simulink model "MIL4L3_SW6_V1_20220211"  (R2018b)
settings: Solver=FixedStepAuto  StartTime=0.0  StopTime=inf  FixedStep=0.001  RelTol=1e-3
PreLoadFcn:
  | A0_MILtest;
undefined symbols (not defined in the file or in its folder): Clb_ICADirect_LaneDisp_StateFive, Clb_ICADirect_LaneDisp_StateFour, Clb_ICADirect_LaneDisp_StateOne, Clb_ICADirect_LaneDisp_StateThree, Clb_ICADirect_LaneDisp_StateTwo, Clb_ICADirect_LaneDisp_StateZero, Clb_ICADirect_LaneDispSW, Clb_ICADirect_TrnLghtsCom_Switch, Clb_ICADirect_TrnLghtsCom_Value, Clb_ICADirect_TrnLghtsCrtl_Inhb, IMAP_Clb_ACU_Driver_Belt, IMAP_Clb_ACU_Driver_Belt_Over, IMAP_Clb_ACU_Passenger_Belt, IMAP_Clb_ACU_Passenger_Belt_Over, IMAP_Clb_ACU_RearLeft_Belt, IMAP_Clb_ACU_RearLeft_Belt_Over, IMAP_Clb_ACU_RearMiddle_Belt, IMAP_Clb_ACU_RearMiddle_Belt_Over, IMAP_Clb_ACU_RearRight_Belt, IMAP_Clb_ACU_RearRight_Belt_Over, IMAP_Clb_AEB_Switch, IMAP_Clb_AEB_Switch_Over, IMAP_Clb_ALC_TLC_Mode, IMAP_Clb_ALC_TLC_Mode_Over, IMAP_Clb_BCM_Battery_Voltage, IMAP_Clb_BCM_Battery_Voltage_Over, IMAP_Clb_BCM_BrakeLamp_State, IMAP_Clb_BCM_BrakeLamp_State_Over, IMAP_Clb_BCM_CHMSL_Status, IMAP_Clb_BCM_CHMSL_Status_Over, IMAP_Clb_BCM_Door_Lock_State, IMAP_Clb_BCM_Door_Lock_State_Over, IMAP_Clb_BCM_FrontWiper_State, IMAP_Clb_BCM_FrontWiper_State_Over, IMAP_Clb_BCM_FrontWiper_Switch, IMAP_Clb_BCM_FrontWiper_Switch_Over, IMAP_Clb_BCM_HazardLamp, IMAP_Clb_BCM_HazardLamp_Over, IMAP_Clb_BCM_HazardLamp_Switch, IMAP_Clb_BCM_HazardLamp_Switch_Over, IMAP_Clb_BCM_HighBeam_State, IMAP_Clb_BCM_HighBeam_State_Over, IMAP_Clb_BCM_Ignition_State, IMAP_Clb_BCM_Ignition_State_Over, IMAP_Clb_BCM_IHBC_Enabled, IMAP_Clb_BCM_IHBC_Enabled_Over, IMAP_Clb_BCM_Left_Light, IMAP_Clb_BCM_Left_Light_Over, IMAP_Clb_BCM_LeftTurn_Switch, IMAP_Clb_BCM_LeftTurn_Switch_Over, IMAP_Clb_BCM_LF_Door_State, IMAP_Clb_BCM_LF_Door_State_Over, IMAP_Clb_BCM_LowBeam_State, IMAP_Clb_BCM_LowBeam_State_Over, IMAP_Clb_BCM_LR_Door_State, IMAP_Clb_BCM_LR_Door_State_Over, IMAP_Clb_BCM_RF_Door_State, IMAP_Clb_BCM_RF_Door_State_Over, IMAP_Clb_BCM_Right_Light, IMAP_Clb_BCM_Right_Light_Over ... (+547)
libraries: CarMaker4SL x2153, simulink x292, dspstat3 x3, canmsglib x2, simulink_extras x1
(part 45 of 52)

== system MIL4L3_SW6_V1_20220211/CarMaker/VehicleControl/Function/LKA/LKAS1/LL/LLOn/LL State Determination (LLStateDet)/LL State Machine Conditions (LLSMCon)/Enable Condition (EnaC)/Vehicle State Condition (VehStateC) ==
  VehStateC_stDACMode : Inport
  VehStateC_bsInInfoSyn : Inport  Port=2
  VehStateC_bsLLClb : Inport  Port=3
  Bus Selector : BusSelector  OutputSignals=bsVehMovInfo.ESC_VehSpd,bsBCMInfo,bsPTState
  Bus Selector1 : BusSelector  OutputSignals=bsLLSMConClb.EnaCClb.LL_MAX_LDWS_SPEED_ENABLE,bsLLSMConClb.EnaCClb.LL_MAX_LKAS_SPEED_ENABLE,bsLLSMConClb.EnaCClb.LL_MIN_LKAS_SPEED_ENABLE
  Emergency Light Enable Condition (EmgcyLghtEC) : Subsystem  Description=|
      | Block Name: Emergency Light Enable Condition
      | Ab.: EmgcyLghtEC
      | No.: 1.1.1.2.1.3
      | Rev: 0.0.1
      | Update Date: 19-3-26
  Gear Enable Condition (GearEC) : Subsystem  Description=|
      | Block Name: Gear Enable Condition
      | Ab.: GearEC
      | No.: 1.1.1.2.1.4
      | Rev: 0.0.1
      | Update Date: 19-3-26
  Vehicle Speed Enable Condition (VehSpdEC) : Subsystem  Description=|
      | Block Name: Vehicle Speed Enable Condition
      | Ab.: VehSpdEC
      | No.: 1.1.1.2.1.1
      | Rev: 0.0.1
      | Update Date: 19-3-26
  Vehicle State Condition Synthesis (VehStateCSyn) : Subsystem  Description=|
      | Block Name: Vehicle State Condition Synthesis
      | Ab.: VehStateCSyn
      | No.: 1.1.1.2.1.5
      | Rev: 0.0.1
      | Update Date: 19-3-26
  VehStateC_stVehStateCSyn : Outport
  wires:
  Vehicle Speed Enable Condition (VehSpdEC)/1(VehSpdEC_stVehSpdECFlg) -> Vehicle State Condition Synthesis (VehStateCSyn)/1(VehStateCSyn_stVehSpdECFlg)  "VEHSTATE_VEHSPEED"
  VehStateC_bsInInfoSyn/1 -> Bus Selector/1
  Gear Enable Condition (GearEC)/1(GearEC_stGearECFlg) -> Vehicle State Condition Synthesis (VehStateCSyn)/3(VehStateCSyn_stGearECFlg)  "VEHSTATE_GEAR"
  Vehicle State Condition Synthesis (VehStateCSyn)/1(VehStateCSyn_stVehStateCSyn) -> VehStateC_stVehStateCSyn/1  "VEHSTATE"
  Bus Selector/1 -> Vehicle Speed Enable Condition (VehSpdEC)/2(VehSpdEC_vVehSpd)  "<ESC_VehSpd>"
  Bus Selector1/1 -> Vehicle Speed Enable Condition (VehSpdEC)/3(VehSpdEC_vLDWVehSpdMax_C)  "<LL_MAX_LDWS_SPEED_ENABLE>"
  Bus Selector1/3 -> Vehicle Speed Enable Condition (VehSpdEC)/5(VehSpdEC_vVehSpdMin_C)  "<LL_MIN_LKAS_SPEED_ENABLE>"
  Bus Selector1/2 -> Vehicle Speed Enable Condition (VehSpdEC)/4(VehSpdEC_vLKAVehSpdMax_C)  "<LL_MAX_LKAS_SPEED_ENABLE>"
  VehStateC_bsLLClb/1 -> Bus Selector1/1
  VehStateC_stDACMode/1 -> Vehicle Speed Enable Condition (VehSpdEC)/1(VehSpdEC_stDACMode)
  Bus Selector/3 -> Gear Enable Condition (GearEC)/1(GearEC_bsTCUState)  "<bsPTState>"
  Bus Selector/2 -> Emergency Light Enable Condition (EmgcyLghtEC)/1(EmgcyLghtEC_bsStLampState)  "<bsBCMInfo>"
  Emergency Light Enable Condition (EmgcyLghtEC)/1(EmgcyLghtEC_stEmgcyLghtECFlg) -> Vehicle State Condition Synthesis (VehStateCSyn)/2(VehStateCSyn_stEmgcyLghtECFlg)  "VEHSTATE_LIGHT"

== system MIL4L3_SW6_V1_20220211/CarMaker/VehicleControl/Function/LKA/LKAS1/LL/LLOn/LL State Determination (LLStateDet)/LL State Machine Conditions (LLSMCon)/Fault Condition (FaultC)/Count_5s1 ==
  SampleTime : Inport
  Enable : EnablePort  StatesWhenEnabling=reset
  Add : Sum
  Constant1 : Constant  Value=5  OutDataTypeStr=uint16
  Memory : Memory  InheritSampleTime=on
  Relational Operator : RelationalOperator  OutDataTypeStr=boolean  RndMeth=Simplest
  Saturation : Saturate  UpperLimit=11  LowerLimit=0
      settings: AttributesFormatString="Min = %<LowerLimit>  Max = %<UpperLimit>"
  Out : Outport  OutputWhenDisabled=reset  InitialOutput=0
      settings: AttributesFormatString=%<OutputWhenDisabled> = %<InitialOutput>
  wires:
  Memory/1 -> Add/1
  Add/1 -> Saturation/1
  SampleTime/1 -> Add/2
  Saturation/1 -> Relational Operator/1, Memory/1
  Relational Operator/1 -> Out/1
  Constant1/1 -> Relational Operator/2

== system MIL4L3_SW6_V1_20220211/CarMaker/VehicleControl/Function/LKA/LKAS1/LL/LLOn/LL State Determination (LLStateDet)/LL State Machine Conditions (LLSMCon)/Fault Condition (FaultC)/Count_5s2 ==
  SampleTime : Inport
  Enable : EnablePort  StatesWhenEnabling=reset
  Add : Sum
  Constant1 : Constant  Value=5  OutDataTypeStr=uint16
  Memory : Memory  InheritSampleTime=on
  Relational Operator : RelationalOperator  OutDataTypeStr=boolean  RndMeth=Simplest
  Saturation : Saturate  UpperLimit=11  LowerLimit=0
      settings: AttributesFormatString="Min = %<LowerLimit>  Max = %<UpperLimit>"
  Out : Outport  OutputWhenDisabled=reset  InitialOutput=0
      settings: AttributesFormatString=%<OutputWhenDisabled> = %<InitialOutput>
  wires:
  Constant1/1 -> Relational Operator/2
  Add/1 -> Saturation/1
  Relational Operator/1 -> Out/1
  SampleTime/1 -> Add/2
  Saturation/1 -> Relational Operator/1, Memory/1
  Memory/1 -> Add/1

== system MIL4L3_SW6_V1_20220211/CarMaker/VehicleControl/Function/LKA/LKAS1/LL/LLOn/LL State Determination (LLStateDet)/LL State Machine Conditions (LLSMCon)/Fault Condition (FaultC)/Count_5s3 ==
  SampleTime : Inport
  Enable : EnablePort  StatesWhenEnabling=reset
  Add : Sum  OutDataTypeStr=single
  Constant1 : Constant  Value=5  OutDataTypeStr=uint16
  Memory : Memory  InheritSampleTime=on
  Relational Operator : RelationalOperator  OutDataTypeStr=boolean  RndMeth=Simplest
  Saturation : Saturate  UpperLimit=11  LowerLimit=0
      settings: AttributesFormatString="Min = %<LowerLimit>  Max = %<UpperLimit>"
  Out : Outport  OutputWhenDisabled=reset  InitialOutput=0
      settings: AttributesFormatString=%<OutputWhenDisabled> = %<InitialOutput>
  wires:
  Saturation/1 -> Relational Operator/1, Memory/1
  Memory/1 -> Add/1
  Add/1 -> Saturation/1
  Relational Operator/1 -> Out/1
  SampleTime/1 -> Add/2
  Constant1/1 -> Relational Operator/2

== system MIL4L3_SW6_V1_20220211/CarMaker/VehicleControl/OMAP/OMAP1/Runnable_OMAP_10ms_sys/OMAP_Module/ACCS_Direct/ACCS_Define/ACC_State_Synthesis(ACC_SS)/If Action Subsystem2/Subsystem ==
  In1 : Inport
  Add : Sum  Inputs=+++  OutDataTypeStr=uint8
  Compare To Constant1 : simulink/Logic and Bit Operations/Compare To Constant  relop===  const=0  OutDataTypeStr=boolean
  Compare To Constant2 : simulink/Logic and Bit Operations/Compare To Constant  relop===  const=1  OutDataTypeStr=boolean
  Compare To Constant3 : simulink/Logic and Bit Operations/Compare To Constant  relop===  const=15  OutDataTypeStr=boolean
  Compare To Constant5 : simulink/Logic and Bit Operations/Compare To Constant  relop===  const=2  OutDataTypeStr=boolean
  Compare To Constant6 : simulink/Logic and Bit Operations/Compare To Constant  relop===  const=3  OutDataTypeStr=boolean
  Gain : Gain  Gain=3
  Gain1 : Gain  Gain=2
  Gain2 : Gain  Gain=15
  Logical Operator1 : Logic  Operator=OR  Inputs=3  AllPortsSameDT=off  OutDataTypeStr=boolean
  Function_Acc_status : Outport
  wires:
  Gain2/1 -> Add/3
  Compare To Constant3/1 -> Gain2/1
  Add/1 -> Function_Acc_status/1
  Gain/1 -> Add/1
  Compare To Constant1/1 -> Logical Operator1/1
  Compare To Constant5/1 -> Gain1/1
  Gain1/1 -> Add/2
  Compare To Constant6/1 -> Logical Operator1/3
  In1/1 -> Compare To Constant2/1, Compare To Constant1/1, Compare To Constant6/1, Compare To Constant5/1, Compare To Constant3/1
  Logical Operator1/1 -> Gain/1
  Compare To Constant2/1 -> Logical Operator1/2

== system MIL4L3_SW6_V1_20220211/CarMaker/VehicleControl/OMAP/OMAP1/Runnable_OMAP_10ms_sys/OMAP_Module/ACCS_Direct/ACCS_Define/ACC_State_Synthesis(ACC_SS)/If Action Subsystem2/Subsystem4 ==
  Chart : Stateflow chart  TreatAsAtomicUnit=on
  TYPE_RAPPORT : Outport
  wires:
  Chart/1(RAPPORT) -> TYPE_RAPPORT/1

== system MIL4L3_SW6_V1_20220211/CarMaker/VehicleControl/OMAP/OMAP1/Runnable_OMAP_10ms_sys/OMAP_Module/ACCS_Direct/ACCS_Define/ACC_State_Synthesis(ACC_SS)/If Action Subsystem3/Subsystem ==
  In1 : Inport
  Constant1 : Constant  Value=6.2  OutDataTypeStr=single
  Constant11 : Constant  Value=6.2  OutDataTypeStr=single
  Switch : Switch  Criteria=u2 > Threshold
  TminDownGear : Outport
  wires:
  Switch/1 -> TminDownGear/1
  Constant1/1 -> Switch/1
  Constant11/1 -> Switch/3
  In1/1 -> Switch/2

== system MIL4L3_SW6_V1_20220211/CarMaker/VehicleControl/OMAP/OMAP1/Runnable_OMAP_10ms_sys/OMAP_Module/ACCS_Direct/ACCS_Define/ACC_State_Synthesis(ACC_SS)/If Action Subsystem3/Subsystem1 ==
  In1 : Inport
  Constant12 : Constant  Value=6.2  OutDataTypeStr=single
  Constant2 : Constant  Value=6.2  OutDataTypeStr=single
  Switch1 : Switch  Criteria=u2 > Threshold
  TminUpGear : Outport
  wires:
  Switch1/1 -> TminUpGear/1
  In1/1 -> Switch1/2
  Constant2/1 -> Switch1/1
  Constant12/1 -> Switch1/3

== system MIL4L3_SW6_V1_20220211/CarMaker/VehicleControl/OMAP/OMAP1/Runnable_OMAP_10ms_sys/OMAP_Module/ACCS_Direct/ACCS_Define/ACC_State_Synthesis(ACC_SS)/If Action Subsystem3/Subsystem2 ==
  In1 : Inport
  In2 : Inport  Port=2
  Constant1 : Constant  Value=2  OutDataTypeStr=uint8
  Constant11 : Constant  OutDataTypeStr=uint8
  Constant2 : Constant  Value=0  OutDataTypeStr=uint8
  Switch : Switch  Criteria=u2 > Threshold
  Switch1 : Switch  Criteria=u2 > Threshold
  StAcvTqWhlPTPotReq : Outport
  wires:
  In1/1 -> Switch1/2
  In2/1 -> Switch/2
  Constant1/1 -> Switch/1
  Constant2/1 -> Switch/3
  Constant11/1 -> Switch1/1
  Switch/1 -> Switch1/3
  Switch1/1 -> StAcvTqWhlPTPotReq/1

== system MIL4L3_SW6_V1_20220211/CarMaker/VehicleControl/OMAP/OMAP1/Runnable_OMAP_10ms_sys/OMAP_Module/ACCS_Direct/ACCS_Define/ACC_State_Synthesis(ACC_SS)/If Action Subsystem3/Subsystem3 ==
  In1 : Inport
  Compare To Constant1 : simulink/Logic and Bit Operations/Compare To Constant  relop===  const=8  OutDataTypeStr=boolean
  Compare To Constant2 : simulink/Logic and Bit Operations/Compare To Constant  relop===  const=7  OutDataTypeStr=boolean
  Constant1 : Constant  Value=7  OutDataTypeStr=uint8
  Logical Operator1 : Logic  Operator=OR  AllPortsSameDT=off  OutDataTypeStr=boolean
  Switch : Switch  Criteria=u2 > Threshold
  Function_Acc_status : Outport
  wires:
  Logical Operator1/1 -> Switch/2
  Switch/1 -> Function_Acc_status/1
  In1/1 -> Switch/3, Compare To Constant1/1, Compare To Constant2/1
  Compare To Constant1/1 -> Logical Operator1/2
  Compare To Constant2/1 -> Logical Operator1/1
  Constant1/1 -> Switch/1

== system MIL4L3_SW6_V1_20220211/CarMaker/VehicleControl/OMAP/OMAP1/Runnable_OMAP_10ms_sys/OMAP_Module/ACCS_Direct/ACCS_Define/ACC_State_Synthesis(ACC_SS)/If Action Subsystem3/Subsystem5 ==
  In1 : Inport
  In2 : Inport  Port=2
  Constant4 : Constant  Value=-4000  OutDataTypeStr=single
  Switch : Switch  Criteria=u2 > Threshold
  PotACCTqReq : Outport
  wires:
  In2/1 -> Switch/2
  In1/1 -> Switch/1
  Constant4/1 -> Switch/3
  Switch/1 -> PotACCTqReq/1

== system MIL4L3_SW6_V1_20220211/CarMaker/VehicleControl/OMAP/OMAP1/Runnable_OMAP_10ms_sys/OMAP_Module/ACCS_Direct/ACCS_Define/ACC_State_Synthesis(ACC_SS)/If Action Subsystem3/Subsystem6 ==
  Chart : Stateflow chart  TreatAsAtomicUnit=on
  TYPE_RAPPORT : Outport
  wires:
  Chart/1(RAPPORT) -> TYPE_RAPPORT/1

== system MIL4L3_SW6_V1_20220211/CarMaker/VehicleControl/OMAP/OMAP1/Runnable_OMAP_10ms_sys/OMAP_Module/ACCS_Direct/ACCS_Define/Human_Machine_Interface(ACC_HMI)/Subsystem9/Subsystem ==
  Bus Creator : BusCreator  Inputs=4
  Constant{,1..3} (4 alike) : Constant  Value=0  OutDataTypeStr=uint16
  Out1 : Outport
  wires:
  Constant/1 -> Bus Creator/1  "ACC_Vehicle_Icon_Display"
  Constant1/1 -> Bus Creator/2  "ACC_Set_Speed_Display"
  Bus Creator/1 -> Out1/1
  Constant2/1 -> Bus Creator/4  "RVVACC_Vehiclespeed_request_type"
  Constant3/1 -> Bus Creator/3  "ACC_DesiredHeadway_Icon_Basic"

== system MIL4L3_SW6_V1_20220211/CarMaker/VehicleControl/OMAP/OMAP1/Runnable_OMAP_10ms_sys/OMAP_Module/ACCS_Direct/ACCS_Define/Human_Machine_Interface(ACC_HMI)/Subsystem9/Subsystem1 ==
  VelocitySet : Inport
  Bus Creator : BusCreator  Inputs=4
  Compare To Constant : simulink/Logic and Bit Operations/Compare To Constant  relop=>  const=10  OutDataTypeStr=boolean
  Constant : Constant  OutDataTypeStr=uint16
  Constant2 : Constant  Value=0  OutDataTypeStr=uint16
  Constant3 : Constant  OutDataTypeStr=uint16
  Constant4 : Constant  OutDataTypeStr=uint16
  Constant5 : Constant  Value=3  OutDataTypeStr=uint16
  Switch : Switch
  Out1 : Outport
  wires:
  Constant3/1 -> Bus Creator/3  "ACC_DesiredHeadway_Icon_Basic"
  Constant2/1 -> Bus Creator/4  "RVVACC_Vehiclespeed_request_type"
  Bus Creator/1 -> Out1/1
  Switch/1 -> Bus Creator/2  "ACC_Set_Speed_Display"
  Constant/1 -> Bus Creator/1  "ACC_Vehicle_Icon_Display"
  VelocitySet/1 -> Compare To Constant/1
  Compare To Constant/1 -> Switch/2
  Constant4/1 -> Switch/1
  Constant5/1 -> Switch/3

== system MIL4L3_SW6_V1_20220211/CarMaker/VehicleControl/OMAP/OMAP1/Runnable_OMAP_10ms_sys/OMAP_Module/ACCS_Direct/ACCS_Define/Human_Machine_Interface(ACC_HMI)/Subsystem9/Subsystem2 ==
  VelocitySet : Inport
  Bus Creator : BusCreator  Inputs=4
  Compare To Constant : simulink/Logic and Bit Operations/Compare To Constant  relop=>  const=10  OutDataTypeStr=boolean
  Constant : Constant  OutDataTypeStr=uint16
  Constant2 : Constant  Value=0  OutDataTypeStr=uint16
  Constant3 : Constant  OutDataTypeStr=uint16
  Constant4 : Constant  Value=2  OutDataTypeStr=uint16
  Constant5 : Constant  Value=3  OutDataTypeStr=uint16
  Switch : Switch
  Out1 : Outport
  wires:
  Constant/1 -> Bus Creator/1  "ACC_Vehicle_Icon_Display"
  Switch/1 -> Bus Creator/2  "ACC_Set_Speed_Display"
  Bus Creator/1 -> Out1/1
  Constant2/1 -> Bus Creator/4  "RVVACC_Vehiclespeed_request_type"
  Constant3/1 -> Bus Creator/3  "ACC_DesiredHeadway_Icon_Basic"
  VelocitySet/1 -> Compare To Constant/1
  Compare To Constant/1 -> Switch/2
  Constant4/1 -> Switch/1
  Constant5/1 -> Switch/3

== system MIL4L3_SW6_V1_20220211/CarMaker/VehicleControl/OMAP/OMAP1/Runnable_OMAP_10ms_sys/OMAP_Module/ACCS_Direct/ACCS_Define/Human_Machine_Interface(ACC_HMI)/Subsystem9/Subsystem3 ==
  Bus Creator : BusCreator  Inputs=4
  Constant : Constant  Value=2  OutDataTypeStr=uint16
  Constant1 : Constant  Value=2  OutDataTypeStr=uint16
  Constant2 : Constant  OutDataTypeStr=uint16
  Constant3 : Constant  OutDataTypeStr=uint16
  Out1 : Outport
  wires:
  Constant3/1 -> Bus Creator/3  "ACC_DesiredHeadway_Icon_Basic"
  Constant2/1 -> Bus Creator/4  "RVVACC_Vehiclespeed_request_type"
  Bus Creator/1 -> Out1/1
  Constant1/1 -> Bus Creator/2  "ACC_Set_Speed_Display"
  Constant/1 -> Bus Creator/1  "ACC_Vehicle_Icon_Display"

== system MIL4L3_SW6_V1_20220211/CarMaker/VehicleControl/OMAP/OMAP1/Runnable_OMAP_10ms_sys/OMAP_Module/ACCS_Direct/ACCS_Define/Human_Machine_Interface(ACC_HMI)/Subsystem9/Subsystem4 ==
  Bus Creator : BusCreator  Inputs=4
  Constant : Constant  Value=2  OutDataTypeStr=uint16
  Constant1 : Constant  Value=4  OutDataTypeStr=uint16
  Constant2 : Constant  OutDataTypeStr=uint16
  Constant3 : Constant  OutDataTypeStr=uint16
  Out1 : Outport
  wires:
  Constant/1 -> Bus Creator/1  "ACC_Vehicle_Icon_Display"
  Constant1/1 -> Bus Creator/2  "ACC_Set_Speed_Display"
  Bus Creator/1 -> Out1/1
  Constant2/1 -> Bus Creator/4  "RVVACC_Vehiclespeed_request_type"
  Constant3/1 -> Bus Creator/3  "ACC_DesiredHeadway_Icon_Basic"

== system MIL4L3_SW6_V1_20220211/CarMaker/VehicleControl/OMAP/OMAP1/Runnable_OMAP_10ms_sys/OMAP_Module/ACCS_Direct/ACCS_Define/Human_Machine_Interface(ACC_HMI)/Subsystem9/Subsystem5 ==
  Bus Creator : BusCreator  Inputs=4
  Constant : Constant  Value=2  OutDataTypeStr=uint16
  Constant1 : Constant  Value=2  OutDataTypeStr=uint16
  Constant2 : Constant  OutDataTypeStr=uint16
  Constant3 : Constant  OutDataTypeStr=uint16
  Out1 : Outport
  wires:
  Constant3/1 -> Bus Creator/3  "ACC_DesiredHeadway_Icon_Basic"
  Constant2/1 -> Bus Creator/4  "RVVACC_Vehiclespeed_request_type"
  Bus Creator/1 -> Out1/1
  Constant1/1 -> Bus Creator/2  "ACC_Set_Speed_Display"
  Constant/1 -> Bus Creator/1  "ACC_Vehicle_Icon_Display"

== system MIL4L3_SW6_V1_20220211/CarMaker/VehicleControl/OMAP/OMAP1/Runnable_OMAP_10ms_sys/OMAP_Module/ACCS_Direct/ACCS_Define/Human_Machine_Interface(ACC_HMI)/Subsystem9/Subsystem6 ==
  Bus Creator : BusCreator  Inputs=4
  Constant : Constant  Value=2  OutDataTypeStr=uint16
  Constant1 : Constant  Value=2  OutDataTypeStr=uint16
  Constant2 : Constant  Value=0  OutDataTypeStr=uint16
  Constant3 : Constant  OutDataTypeStr=uint16
  Out1 : Outport
  wires:
  Constant/1 -> Bus Creator/1  "ACC_Vehicle_Icon_Display"
  Constant1/1 -> Bus Creator/2  "ACC_Set_Speed_Display"
  Bus Creator/1 -> Out1/1
  Constant2/1 -> Bus Creator/4  "RVVACC_Vehiclespeed_request_type"
  Constant3/1 -> Bus Creator/3  "ACC_DesiredHeadway_Icon_Basic"

== system MIL4L3_SW6_V1_20220211/CarMaker/VehicleControl/OMAP/OMAP1/Runnable_OMAP_10ms_sys/OMAP_Module/ACCS_Direct/ACCS_Define/Human_Machine_Interface(ACC_HMI)/Subsystem9/Subsystem7 ==
  Bus Creator : BusCreator  Inputs=4
  Constant : Constant  Value=2  OutDataTypeStr=uint16
  Constant1 : Constant  Value=2  OutDataTypeStr=uint16
  Constant2 : Constant  Value=0  OutDataTypeStr=uint16
  Constant3 : Constant  OutDataTypeStr=uint16
  Out1 : Outport
  wires:
  Constant3/1 -> Bus Creator/3  "ACC_DesiredHeadway_Icon_Basic"
  Constant2/1 -> Bus Creator/4  "RVVACC_Vehiclespeed_request_type"
  Bus Creator/1 -> Out1/1
  Constant1/1 -> Bus Creator/2  "ACC_Set_Speed_Display"
  Constant/1 -> Bus Creator/1  "ACC_Vehicle_Icon_Display"

== system MIL4L3_SW6_V1_20220211/CarMaker/VehicleControl/OMAP/OMAP1/Runnable_OMAP_10ms_sys/OMAP_Module/ACCS_Direct/ACCS_Define/Human_Machine_Interface(ACC_HMI)/Subsystem9/Subsystem8 ==
  Bus Creator : BusCreator  Inputs=4
  Constant : Constant  Value=3  OutDataTypeStr=uint16
  Constant1 : Constant  Value=3  OutDataTypeStr=uint16
  Constant2 : Constant  Value=0  OutDataTypeStr=uint16
  Constant3 : Constant  Value=0  OutDataTypeStr=uint16
  Out1 : Outport
  wires:
  Constant/1 -> Bus Creator/1  "ACC_Vehicle_Icon_Display"
  Constant1/1 -> Bus Creator/2  "ACC_Set_Speed_Display"
  Bus Creator/1 -> Out1/1
  Constant2/1 -> Bus Creator/4  "RVVACC_Vehiclespeed_request_type"
  Constant3/1 -> Bus Creator/3  "ACC_DesiredHeadway_Icon_Basic"

== system MIL4L3_SW6_V1_20220211/CarMaker/VehicleControl/OMAP/OMAP1/Runnable_OMAP_10ms_sys/OMAP_Module/ACCS_Direct/ACCS_Define/Human_Machine_Interface(ACC_HMI)/Text_PopUp/ Radar_Blocked ==
  In1 : Inport
  Chart : Stateflow chart  TreatAsAtomicUnit=on
  Compare To Constant1 : simulink/Logic and Bit Operations/Compare To Constant  relop=~=  const=6  OutDataTypeStr=boolean
  Compare To Constant15 : simulink/Logic and Bit Operations/Compare To Constant  relop===  const=6  OutDataTypeStr=boolean
  Logical Operator : Logic  AllPortsSameDT=off  OutDataTypeStr=boolean
  Unit Delay : UnitDelay  SampleTime=-1
  Out1 : Outport
  wires:
  In1/1 -> Compare To Constant15/1, Unit Delay/1
  Compare To Constant15/1 -> Logical Operator/2
  Unit Delay/1 -> Compare To Constant1/1
  Compare To Constant1/1 -> Logical Operator/1
  Logical Operator/1 -> Chart/1(data)
  Chart/1(Value) -> Out1/1

== system MIL4L3_SW6_V1_20220211/CarMaker/VehicleControl/OMAP/OMAP1/Runnable_OMAP_10ms_sys/OMAP_Module/ACCS_Direct/ACCS_Define/Human_Machine_Interface(ACC_HMI)/Text_PopUp/ACC_Activation_Unsatisfied ==
  In1 : Inport
  In2 : Inport  Port=2
  Chart : Stateflow chart  TreatAsAtomicUnit=on
  Compare To Constant17 : simulink/Logic and Bit Operations/Compare To Constant  relop===  const=2  OutDataTypeStr=boolean
  Logical Operator8 : Logic  AllPortsSameDT=off  OutDataTypeStr=boolean
  Out1 : Outport
  wires:
  Compare To Constant17/1 -> Logical Operator8/1
  In2/1 -> Logical Operator8/2
  Logical Operator8/1 -> Chart/1(data)
  In1/1 -> Compare To Constant17/1
  Chart/1(Value) -> Out1/1

== system MIL4L3_SW6_V1_20220211/CarMaker/VehicleControl/OMAP/OMAP1/Runnable_OMAP_10ms_sys/OMAP_Module/ACCS_Direct/ACCS_Define/Human_Machine_Interface(ACC_HMI)/Text_PopUp/ACC_Active ==
  In1 : Inport
  Chart : Stateflow chart  TreatAsAtomicUnit=on
  Compare To Constant12 : simulink/Logic and Bit Operations/Compare To Constant  relop===  const=3  OutDataTypeStr=boolean
  Compare To Constant13 : simulink/Logic and Bit Operations/Compare To Constant  relop===  const=4  OutDataTypeStr=boolean
  Logical Operator6 : Logic  AllPortsSameDT=off  OutDataTypeStr=boolean
  Unit Delay1 : UnitDelay  SampleTime=-1
  Out1 : Outport
  wires:
  Unit Delay1/1 -> Compare To Constant12/1
  In1/1 -> Unit Delay1/1, Compare To Constant13/1
  Compare To Constant12/1 -> Logical Operator6/1
  Compare To Constant13/1 -> Logical Operator6/2
  Logical Operator6/1 -> Chart/1(data)
  Chart/1(Value) -> Out1/1

== system MIL4L3_SW6_V1_20220211/CarMaker/VehicleControl/OMAP/OMAP1/Runnable_OMAP_10ms_sys/OMAP_Module/ACCS_Direct/ACCS_Define/Human_Machine_Interface(ACC_HMI)/Text_PopUp/ACC_Canceled ==
  In1 : Inport
  Chart : Stateflow chart  TreatAsAtomicUnit=on
  Compare To Constant1 : simulink/Logic and Bit Operations/Compare To Constant  relop===  const=2  OutDataTypeStr=boolean
  Compare To Constant2 : simulink/Logic and Bit Operations/Compare To Constant  relop===  const=3  OutDataTypeStr=boolean
  Compare To Constant23 : simulink/Logic and Bit Operations/Compare To Constant  relop===  const=4  OutDataTypeStr=boolean
  Compare To Constant3 : simulink/Logic and Bit Operations/Compare To Constant  relop===  const=7  OutDataTypeStr=boolean
  Compare To Constant4 : simulink/Logic and Bit Operations/Compare To Constant  relop===  const=6  OutDataTypeStr=boolean
  Compare To Constant5 : simulink/Logic and Bit Operations/Compare To Constant  relop===  const=2  OutDataTypeStr=boolean
  Compare To Constant6 : simulink/Logic and Bit Operations/Compare To Constant  relop===  const=3  OutDataTypeStr=boolean
  Compare To Constant7 : simulink/Logic and Bit Operations/Compare To Constant  relop===  const=5  OutDataTypeStr=boolean
  Logical Operator1 : Logic  Operator=OR  Inputs=3  AllPortsSameDT=off  OutDataTypeStr=boolean
  Logical Operator16 : Logic  AllPortsSameDT=off  OutDataTypeStr=boolean
  Logical Operator2 : Logic  Operator=OR  AllPortsSameDT=off  OutDataTypeStr=boolean
  Logical Operator3 : Logic  Operator=OR  AllPortsSameDT=off  OutDataTypeStr=boolean
  Logical Operator4 : Logic  AllPortsSameDT=off  OutDataTypeStr=boolean
  Logical Operator5 : Logic  Operator=OR  AllPortsSameDT=off  OutDataTypeStr=boolean
  Unit Delay1 : UnitDelay  SampleTime=-1
  Unit Delay5 : UnitDelay  SampleTime=-1
  Out1 : Outport
  wires:
  Compare To Constant1/1 -> Logical Operator1/1
  Compare To Constant23/1 -> Logical Operator16/1
  Logical Operator16/1 -> Logical Operator2/1
  Chart/1(Value) -> Out1/1
  Unit Delay5/1 -> Compare To Constant23/1
  Compare To Constant2/1 -> Logical Operator1/2
  Compare To Constant3/1 -> Logical Operator1/3
  Logical Operator1/1 -> Logical Operator16/2
  Compare To Constant5/1 -> Logical Operator3/1
  Compare To Constant7/1 -> Logical Operator5/1
  In1/1 -> Compare To Constant6/1, Compare To Constant5/1, Unit Delay1/1, Compare To Constant3/1, Compare To Constant2/1, Compare To Constant1/1, Unit Delay5/1
  Unit Delay1/1 -> Compare To Constant4/1, Compare To Constant7/1
  Compare To Constant6/1 -> Logical Operator3/2
  Logical Operator3/1 -> Logical Operator4/2
  Logical Operator4/1 -> Logical Operator2/2
  Logical Operator2/1 -> Chart/1(data)
  Compare To Constant4/1 -> Logical Operator5/2
  Logical Operator5/1 -> Logical Operator4/1

== system MIL4L3_SW6_V1_20220211/CarMaker/VehicleControl/OMAP/OMAP1/Runnable_OMAP_10ms_sys/OMAP_Module/ACCS_Direct/ACCS_Define/Human_Machine_Interface(ACC_HMI)/Text_PopUp/ACC_Fault ==
  In1 : Inport
  Chart : Stateflow chart  TreatAsAtomicUnit=on
  Compare To Constant1 : simulink/Logic and Bit Operations/Compare To Constant  relop=~=  const=15  OutDataTypeStr=boolean
  Compare To Constant15 : simulink/Logic and Bit Operations/Compare To Constant  relop===  const=15  OutDataTypeStr=boolean
  Logical Operator : Logic  AllPortsSameDT=off  OutDataTypeStr=boolean
  Unit Delay : UnitDelay  SampleTime=-1
  Out1 : Outport
  wires:
  Logical Operator/1 -> Chart/1(data)
  In1/1 -> Compare To Constant15/1, Unit Delay/1
  Compare To Constant1/1 -> Logical Operator/1
  Compare To Constant15/1 -> Logical Operator/2
  Unit Delay/1 -> Compare To Constant1/1
  Chart/1(Value) -> Out1/1

== system MIL4L3_SW6_V1_20220211/CarMaker/VehicleControl/OMAP/OMAP1/Runnable_OMAP_10ms_sys/OMAP_Module/ACCS_Direct/ACCS_Define/Human_Machine_Interface(ACC_HMI)/Text_PopUp/ACC_OFF ==
  In1 : Inport
  In2 : Inport  Port=2
  Chart : Stateflow chart  TreatAsAtomicUnit=on
  Compare To Constant1 : simulink/Logic and Bit Operations/Compare To Constant  relop===  const=1  OutDataTypeStr=boolean
  Compare To Constant10 : simulink/Logic and Bit Operations/Compare To Constant  relop===  const=8  OutDataTypeStr=boolean
  Compare To Constant2 : simulink/Logic and Bit Operations/Compare To Constant  relop=~=  const=0  OutDataTypeStr=boolean
  Compare To Constant3 : simulink/Logic and Bit Operations/Compare To Constant  relop=~=  const=15  OutDataTypeStr=boolean
  Compare To Constant4 : simulink/Logic and Bit Operations/Compare To Constant  relop=~=  const=1  OutDataTypeStr=boolean
  Compare To Constant5 : simulink/Logic and Bit Operations/Compare To Constant  relop=~=  const=8  OutDataTypeStr=boolean
  Compare To Constant6 : simulink/Logic and Bit Operations/Compare To Constant  relop===  const=0  OutDataTypeStr=boolean
  Compare To Constant7 : simulink/Logic and Bit Operations/Compare To Constant  relop===  const=1  OutDataTypeStr=boolean
  Compare To Constant8 : simulink/Logic and Bit Operations/Compare To Constant  relop===  const=4  OutDataTypeStr=boolean
  Logical Operator1 : Logic  Inputs=4  AllPortsSameDT=off  OutDataTypeStr=boolean
  Logical Operator2 : Logic  AllPortsSameDT=off  OutDataTypeStr=boolean
  Logical Operator3 : Logic  AllPortsSameDT=off  OutDataTypeStr=boolean
  Logical Operator4 : Logic  Operator=OR  AllPortsSameDT=off  OutDataTypeStr=boolean
  Logical Operator5 : Logic  AllPortsSameDT=off  OutDataTypeStr=boolean
  Unit Delay1 : UnitDelay  SampleTime=-1
  Unit Delay2 : UnitDelay  SampleTime=-1
  Unit Delay6 : UnitDelay  SampleTime=-1
  Out1 : Outport
  wires:
  Unit Delay6/1 -> Compare To Constant8/1
  Logical Operator3/1 -> Logical Operator4/1
  Compare To Constant10/1 -> Logical Operator3/2
  Compare To Constant8/1 -> Logical Operator3/1
  Chart/1(Value) -> Out1/1
  Unit Delay1/1 -> Compare To Constant5/1, Compare To Constant4/1, Compare To Constant3/1, Compare To Constant2/1
  Compare To Constant1/1 -> Logical Operator2/2
  Compare To Constant2/1 -> Logical Operator1/1
  In1/1 -> Unit Delay1/1, Compare To Constant1/1, Compare To Constant10/1, Unit Delay6/1
  Compare To Constant3/1 -> Logical Operator1/2
  Compare To Constant4/1 -> Logical Operator1/3
  Compare To Constant5/1 -> Logical Operator1/4
  Logical Operator1/1 -> Logical Operator2/1
  Logical Operator2/1 -> Logical Operator4/2
  Logical Operator4/1 -> Chart/1(data)
  In2/1 -> Unit Delay2/1, Compare To Constant6/1
  Compare To Constant7/1 -> Logical Operator5/1
  Compare To Constant6/1 -> Logical Operator5/2
  Unit Delay2/1 -> Compare To Constant7/1
  Logical Operator5/1 -> Chart/2(data1)

== system MIL4L3_SW6_V1_20220211/CarMaker/VehicleControl/OMAP/OMAP1/Runnable_OMAP_10ms_sys/OMAP_Module/ACCS_Direct/ACCS_Define/Human_Machine_Interface(ACC_HMI)/Text_PopUp/ACC_ON ==
  In1 : Inport
  In2 : Inport  Port=2
  ACCICA_Flag : Inport  Port=3
  Chart : Stateflow chart  TreatAsAtomicUnit=on
  Compare To Constant{1..2,6,9} (4 alike) : simulink/Logic and Bit Operations/Compare To Constant  relop===  const=1  OutDataTypeStr=boolean
  Compare To Constant10 : simulink/Logic and Bit Operations/Compare To Constant  relop=~=  const=1  OutDataTypeStr=boolean
  Compare To Constant11 : simulink/Logic and Bit Operations/Compare To Constant  relop=~=  const=15  OutDataTypeStr=boolean
  Compare To Constant14 : simulink/Logic and Bit Operations/Compare To Constant  relop===  const=3  OutDataTypeStr=boolean
  Compare To Constant3 : simulink/Logic and Bit Operations/Compare To Constant  relop===  const=2  OutDataTypeStr=boolean
  Compare To Constant4 : simulink/Logic and Bit Operations/Compare To Constant  relop=~=  const=1  OutDataTypeStr=boolean
  Compare To Constant5 : simulink/Logic and Bit Operations/Compare To Constant  relop=~=  const=0  OutDataTypeStr=boolean
  Compare To Constant7 : simulink/Logic and Bit Operations/Compare To Constant  relop===  const=0  OutDataTypeStr=boolean
  Compare To Constant8 : simulink/Logic and Bit Operations/Compare To Constant  relop===  const=0  OutDataTypeStr=boolean
  Logical Operator : Logic  Inputs=3  AllPortsSameDT=off  OutDataTypeStr=boolean
  Logical Operator1 : Logic  AllPortsSameDT=off  OutDataTypeStr=boolean
  Logical Operator2 : Logic  AllPortsSameDT=off  OutDataTypeStr=boolean
  Logical Operator3 : Logic  AllPortsSameDT=off  OutDataTypeStr=boolean
  Logical Operator4 : Logic  Operator=OR  AllPortsSameDT=off  OutDataTypeStr=boolean
  Logical Operator5 : Logic  Inputs=3  AllPortsSameDT=off  OutDataTypeStr=boolean
  Logical Operator9 : Logic  Operator=OR  AllPortsSameDT=off  OutDataTypeStr=boolean
  Unit Delay : UnitDelay  SampleTime=-1
  Unit Delay1 : UnitDelay  SampleTime=-1
  Unit Delay2 : UnitDelay  SampleTime=-1
  Out1 : Outport
  wires:
  Compare To Constant14/1 -> Logical Operator9/2
  Compare To Constant1/1 -> Logical Operator/1
  Logical Operator/1 -> Chart/1(data)
  Logical Operator9/1 -> Logical Operator/2
  Unit Delay/1 -> Compare To Constant1/1
  Compare To Constant3/1 -> Logical Operator9/1
  Chart/1(Value) -> Out1/1
  In2/1 -> Compare To Constant4/1, Unit Delay1/1
  Unit Delay1/1 -> Compare To Constant2/1
  Compare To Constant2/1 -> Logical Operator1/1
  Compare To Constant4/1 -> Logical Operator1/2
  Logical Operator4/1 -> Chart/2(data1)
  In1/1 -> Compare To Constant11/1, Compare To Constant10/1, Compare To Constant5/1, Compare To Constant14/1, Compare To Constant3/1, Unit Delay/1
  Logical Operator5/1 -> Logical Operator2/2
  ACCICA_Flag/1 -> Compare To Constant8/1, Compare To Constant9/1, Compare To Constant7/1, Unit Delay2/1
  Unit Delay2/1 -> Compare To Constant6/1
  Compare To Constant6/1 -> Logical Operator3/1
  Compare To Constant7/1 -> Logical Operator3/2
  Logical Operator3/1 -> Logical Operator2/1
  Logical Operator2/1 -> Chart/3(data2)
  Compare To Constant8/1 -> Logical Operator/3
  Logical Operator1/1 -> Logical Operator4/2
  Compare To Constant9/1 -> Logical Operator4/1
  Compare To Constant5/1 -> Logical Operator5/1
  Compare To Constant10/1 -> Logical Operator5/2
  Compare To Constant11/1 -> Logical Operator5/3

== system MIL4L3_SW6_V1_20220211/CarMaker/VehicleControl/OMAP/OMAP1/Runnable_OMAP_10ms_sys/OMAP_Module/ACCS_Direct/ACCS_Define/Human_Machine_Interface(ACC_HMI)/Text_PopUp/ACC_go_request ==
  In1 : Inport
  Compare To Constant1 : simulink/Logic and Bit Operations/Compare To Constant  relop===  const=1  OutDataTypeStr=boolean
  <GoRequest> : Outport
  wires:
  In1/1 -> Compare To Constant1/1
  Compare To Constant1/1 -> <GoRequest>/1

== system MIL4L3_SW6_V1_20220211/CarMaker/VehicleControl/OMAP/OMAP1/Runnable_OMAP_10ms_sys/OMAP_Module/ACCS_Direct/ACCS_Define/Human_Machine_Interface(ACC_HMI)/Text_PopUp/Please_Take_Over_the_Car ==
  In1 : Inport
  Chart1 : Stateflow chart  TreatAsAtomicUnit=on
  Compare To Constant1 : simulink/Logic and Bit Operations/Compare To Constant  relop===  const=6  OutDataTypeStr=boolean
  Compare To Constant18 : simulink/Logic and Bit Operations/Compare To Constant  relop===  const=6  OutDataTypeStr=boolean
  Compare To Constant19 : simulink/Logic and Bit Operations/Compare To Constant  relop===  const=4  OutDataTypeStr=boolean
  Compare To Constant2 : simulink/Logic and Bit Operations/Compare To Constant  relop=~=  const=6  OutDataTypeStr=boolean
  Logical Operator1 : Logic  AllPortsSameDT=off  OutDataTypeStr=boolean
  Logical Operator7 : Logic  AllPortsSameDT=off  OutDataTypeStr=boolean
  Unit Delay1 : UnitDelay  SampleTime=-1
  Unit Delay2 : UnitDelay  SampleTime=-1
  Out1 : Outport
  wires:
  Logical Operator7/1 -> Chart1/1(IN)
  Compare To Constant18/1 -> Logical Operator7/2
  Unit Delay2/1 -> Compare To Constant19/1
  Compare To Constant19/1 -> Logical Operator7/1
  Chart1/1(Value) -> Out1/1
  Unit Delay1/1 -> Compare To Constant1/1
  Compare To Constant1/1 -> Logical Operator1/1
  Compare To Constant2/1 -> Logical Operator1/2
  Logical Operator1/1 -> Chart1/2(OUT)
  In1/1 -> Unit Delay1/1, Compare To Constant2/1, Compare To Constant18/1, Unit Delay2/1

== system MIL4L3_SW6_V1_20220211/CarMaker/VehicleControl/OMAP/OMAP1/Runnable_OMAP_10ms_sys/OMAP_Module/ACCS_Direct/ACCS_Define/Human_Machine_Interface(ACC_HMI)/Text_PopUp/Please_Take_Over_the_Car_immediataly ==
  ESC_DecTar : Inport
  BRAKE_RELEASED_FAILSAFE1 : Constant  Value=0  OutDataTypeStr=boolean
  Chart1 : Stateflow chart  TreatAsAtomicUnit=on
  Out1 : Outport
  wires:
  Chart1/1(Value) -> Out1/1
  ESC_DecTar/1 -> Chart1/1(ESC_DecTar)
  BRAKE_RELEASED_FAILSAFE1/1 -> Chart1/2(BRAKE_RELEASED_FAILSAFE)

== system MIL4L3_SW6_V1_20220211/CarMaker/VehicleControl/OMAP/OMAP1/Runnable_OMAP_10ms_sys/OMAP_Module/ICA_Direct_G59/ICA_Define/Subsystem1/Dspl/DsplPrcs ==
  note: 0是运动，1是静止
  note: 0是脱手，1是不脱手
  DsplPrcs_stStWhlHld : Inport
  DsplPrcs_stTkOvStChk : Inport  Port=2
  DsplPrcs_facmL0Ql : Inport  Port=3
  DsplPrcs_facmR0Ql : Inport  Port=4
  DsplPrcs_facmL0Type : Inport  Port=5
  DsplPrcs_facmR0Type : Inport  Port=6
  DsplPrcs_stTHState : Inport  Port=7
  DsplPrcs_bsFromFMCMsg : Inport  Port=8
  DsplPrcs_stTHFKeyState : Inport  Port=9
  DsplPrcs_stVehSty : Inport  Port=10
  DsplPrcs_tfAddVocCmd : Inport  Port=11
  DsplPrcs_stSWALimFlg : Inport  Port=12
  DsplPrcs_dDgrdIconWarnflag : Inport  Port=13
  DsplPrcs_stturn_lightState : Inport  Port=14
  DsplPrcs_stTLC_ALCmodeSW : Inport  Port=15
  DsplPrcs_stLC_SpdCndtFlg : Inport  Port=16
  DsplPrcs_dHndOffTxtWarnnum : Inport  Port=17
  DsplPrcs_dDgrdVocWarnDurnum : Inport  Port=18
  DsplPrcs_dHndOffVocWarnnum : Inport  Port=19
  DsplPrcs_dTxtLimnum : Inport  Port=20
  DsplPrcs_dDgrdIconWarnHiDurnum : Inport  Port=21
  DsplPrcs_dDgrdIconWarnLoDurnum : Inport  Port=22
  DsplPrcs_tiSWALimFlgDetnum : Inport  Port=23
  Bus Creator1 : BusCreator  Inputs=4
  Bus Selector : BusSelector  OutputSignals=stLaneDspl,stL0DispType,stR0DispType
  Bus Selector1 : BusSelector  OutputSignals=ACC_State
  Bus Selector2 : BusSelector  OutputSignals=Icon_stICAIcon,Icon_stHWAmode
  Data Type Conversion1 : DataTypeConversion  OutDataTypeStr=uint16
  Icon : Subsystem
  Lane : Subsystem
  Txt : Subsystem
  Voc : Subsystem
  DsplPrcs_stTxtDspl : Outport
  DsplPrcs_stICAIcon : Outport  Port=2
  DsplPrcs_stLaneDspl : Outport  Port=3
  DsplPrcs_stL0DispType : Outport  Port=4
  DsplPrcs_stR0DispType : Outport  Port=5
  DsplPrcs_stVocDspl : Outport  Port=6
  DsplPrcs_stHWAmode : Outport  Port=7
  DsplPrcs_bsMon : Outport  Port=8
  wires:
  DsplPrcs_stTHFKeyState/1 -> Txt/4(Txt_stTHFKeyState)
  Txt/1(Txt_stTxtDspl) -> DsplPrcs_stTxtDspl/1
  DsplPrcs_stTHState/1 -> Voc/2(Voc_stTHState), Lane/1(Lane_stTHState), Icon/1(Icon_stTHState), Txt/6(Txt_stTHState)
  Icon/1(Icon_stIconDspl) -> Bus Creator1/2, Bus Selector2/1  "stIconDspl"
  Lane/1(Lane_stLaneDspl) -> Bus Selector/1, Bus Creator1/3  "Vehicle_Lane_Display"
  Txt/2(Txt_bsMon) -> Bus Creator1/1  "ICA_HMI_Txt_Mon"
  Bus Creator1/1 -> DsplPrcs_bsMon/1
  DsplPrcs_stStWhlHld/1 -> Txt/1(Txt_stStWhlHld), Voc/1(Voc_stStWhlHld)
  DsplPrcs_dHndOffTxtWarnnum/1 -> Txt/5(Txt_dHndOffTxtWarnnum)
  Voc/1(Voc_stVocDspl) -> DsplPrcs_stVocDspl/1, Bus Creator1/4  "Hands_off_warning"
  DsplPrcs_dHndOffVocWarnnum/1 -> Voc/4(Voc_dHndOffVocWarnnum)
  DsplPrcs_dDgrdVocWarnDurnum/1 -> Voc/3(Voc_dDgrdVocWarnDurnum)
  DsplPrcs_bsFromFMCMsg/1 -> Bus Selector1/1, Txt/3(Txt_bsFromFMCMsg)
  Data Type Conversion1/1 -> Icon/2(Icon_stACCState)
  Bus Selector1/1 -> Data Type Conversion1/1  "<ACC_State>"
  DsplPrcs_dTxtLimnum/1 -> Txt/7(Txt_dTxtLimnum)
  DsplPrcs_facmL0Ql/1 -> Lane/3(Lane_facmL0Ql)
  DsplPrcs_facmR0Ql/1 -> Lane/4(Lane_facmR0Ql)
  DsplPrcs_stVehSty/1 -> Txt/2(Txt_stVehSty), Lane/2(Lane_stVehSty), Voc/5(Voc_stVehSty)
  DsplPrcs_tfAddVocCmd/1 -> Txt/11(Txt_tfAddVocCmd)
  DsplPrcs_dDgrdIconWarnHiDurnum/1 -> Icon/3(Icon_dDgrdIconWarnHiDurnum)
  DsplPrcs_dDgrdIconWarnLoDurnum/1 -> Icon/4(Icon_dDgrdIconWarnLoDurnum)
  DsplPrcs_dDgrdIconWarnflag/1 -> Icon/5(Icon_dDgrdIconWarnflag)
  DsplPrcs_stSWALimFlg/1 -> Txt/8(Txt_stSWALimFlg)
  DsplPrcs_tiSWALimFlgDetnum/1 -> Txt/9(Txt_tiSWALimFlgDetnum)
  DsplPrcs_facmL0Type/1 -> Lane/5(Lane_facmL0Type)
  DsplPrcs_facmR0Type/1 -> Lane/6(Lane_facmR0Type)
  Bus Selector/1 -> DsplPrcs_stLaneDspl/1  "<stLaneDspl>"
  Bus Selector/2 -> DsplPrcs_stL0DispType/1  "<stL0DispType>"
  Bus Selector/3 -> DsplPrcs_stR0DispType/1  "<stR0DispType>"
  DsplPrcs_stturn_lightState/1 -> Lane/7(Lane_stturn_lightState)
  DsplPrcs_stTLC_ALCmodeSW/1 -> Lane/8(Lane_stTLC_ALCmodeSW)
  DsplPrcs_stTkOvStChk/1 -> Txt/10(Txt_stTkOvStChk), Icon/6(Icon_stTLC_ALCmodeSW), Lane/9(Lane_stTkOvStChk)
  DsplPrcs_stLC_SpdCndtFlg/1 -> Icon/7(Icon_stLC_SpdCndtFlg)
  Bus Selector2/2 -> DsplPrcs_stHWAmode/1  "<Icon_stHWAmode>"
  Bus Selector2/1 -> DsplPrcs_stICAIcon/1  "<Icon_stICAIcon>"

== system MIL4L3_SW6_V1_20220211/CarMaker/VehicleControl/OMAP/OMAP1/Runnable_OMAP_10ms_sys/OMAP_Module/ICA_Direct_G59/ICA_Define/Subsystem1/Dspl/TimePrcs ==
  note: 降级图标闪烁的单次点亮时间，1.3s
  note: 文字提示的最长显示时间，3s
  note: 方向盘转角限幅报警的时间阈值
  note: 功能降级声音提示时长，0.5s
  note: 降级图标闪烁的单次熄灭时间，0.2s
  TimePrcs_tiHndOffTxtWarnT_C : Inport
  TimePrcs_tiDgrdVocWarnDurT_C : Inport  Port=2
  TimePrcs_tiHndOffVocWarnT_C : Inport  Port=3
  TimePrcs_tiTxtLimT_C : Inport  Port=4
  TimePrcs_tiDgrdIconWarnHiDurT_C : Inport  Port=5
  TimePrcs_tiDgrdIconWarnLoDurT_C : Inport  Port=6
  TimePrcs_tiSWALimFlgDetT_C : Inport  Port=7
  TimePrcs_tiCalcPer_C : Inport  Port=8
  Divide{,1..6} (7 alike) : Product  Inputs=*/  OutDataTypeStr=uint16
  Switch : Switch  Criteria=u2 ~= 0  OutDataTypeStr=single
  constant : Constant  Value=0.01  OutDataTypeStr=single
  TimePrcs_dHndOffTxtWarnnum : Outport
  TimePrcs_dDgrdVocWarnDurnum : Outport  Port=2
  TimePrcs_dHndOffVocWarnnum : Outport  Port=3
  TimePrcs_dTxtLimnum : Outport  Port=4
  TimePrcs_dDgrdIconWarnHiDurnum : Outport  Port=5
  TimePrcs_dDgrdIconWarnLoDurnum : Outport  Port=6
  TimePrcs_tiSWALimFlgDetnum : Outport  Port=7
  wires:
  Divide/1 -> TimePrcs_dHndOffTxtWarnnum/1
  TimePrcs_tiCalcPer_C/1 -> Switch/1, Switch/2
  constant/1 -> Switch/3
  TimePrcs_tiHndOffTxtWarnT_C/1 -> Divide/1
  Switch/1 -> Divide5/2, Divide4/2, Divide3/2, Divide2/2, Divide1/2, Divide/2, Divide6/2
  TimePrcs_tiDgrdVocWarnDurT_C/1 -> Divide1/1
  TimePrcs_tiHndOffVocWarnT_C/1 -> Divide2/1
  TimePrcs_tiTxtLimT_C/1 -> Divide3/1
  Divide1/1 -> TimePrcs_dDgrdVocWarnDurnum/1
  Divide2/1 -> TimePrcs_dHndOffVocWarnnum/1
  Divide3/1 -> TimePrcs_dTxtLimnum/1
  TimePrcs_tiDgrdIconWarnHiDurT_C/1 -> Divide4/1
  Divide4/1 -> TimePrcs_dDgrdIconWarnHiDurnum/1
  TimePrcs_tiDgrdIconWarnLoDurT_C/1 -> Divide5/1
  Divide5/1 -> TimePrcs_dDgrdIconWarnLoDurnum/1
  Divide6/1 -> TimePrcs_tiSWALimFlgDetnum/1
  TimePrcs_tiSWALimFlgDetT_C/1 -> Divide6/1

== system MIL4L3_SW6_V1_20220211/CarMaker/VehicleControl/OMAP/OMAP1/Runnable_OMAP_10ms_sys/OMAP_Module/ICA_Direct_G59/ICA_Define/Subsystem1/Subsystem/Subsystem ==
  HiDurnum : Inport
  LoDurnum : Inport  Port=2
  Add : Sum
  Constant1 : Constant  Value=0  OutDataTypeStr=uint16
  Constant8 : Constant  OutDataTypeStr=uint16
  Count : Terminator
  Relational Operator1 : RelationalOperator  Operator=<=  OutDataTypeStr=boolean  RndMeth=Nearest
  Relational Operator2 : RelationalOperator  Operator=<=  OutDataTypeStr=boolean  RndMeth=Nearest
  Sum : Sum  OutDataTypeStr=Inherit: Inherit via back propagation  InputSameDT=on
  Unit Delay1 : UnitDelay  SampleTime=-1
  Unit Delay2 : UnitDelay  SampleTime=-1
  reset switch1 : Switch  Criteria=u2 ~= 0  Threshold=1  OutDataTypeStr=Inherit: Inherit via back propagation  InputSameDT=on
  Signal : Outport
  wires:
  Unit Delay2/1 -> Sum/2
  HiDurnum/1 -> Relational Operator2/2, Add/1
  Unit Delay1/1 -> [reset]
  Add/1 -> Relational Operator1/1
  [reset] -> reset switch1/2
  Constant8/1 -> Sum/1
  Relational Operator1/1 -> Unit Delay1/1
  reset switch1/1 -> Count/1, Relational Operator2/1, Relational Operator1/2, Unit Delay2/1
  Constant1/1 -> reset switch1/1
  LoDurnum/1 -> Add/2
  Relational Operator2/1 -> Signal/1
  Sum/1 -> reset switch1/3

== system MIL4L3_SW6_V1_20220211/CarMaker/VehicleControl/Function/LKA/LKAS1/LL/LL Inputs Mapping/bsLaneInfo/LanesReconstruct /RoadSide Offset/CrvDvtR0C0/Average Filter (AvrgFlt)1 ==
  In : Inport
  PtsNum : Inport  Port=2
  Abs : Abs
  Add1 : Sum  AccumDataTypeStr=single  OutDataTypeStr=single
  Add2 : Sum  Inputs=-+
  Add3 : Sum  Inputs=+-  AccumDataTypeStr=single  OutDataTypeStr=single
  Compare To Constant : simulink/Logic and Bit Operations/Compare To Constant  relop=>  const=0.5  OutDataTypeStr=boolean
  Constant : Constant  OutDataTypeStr=single
  Constant1 : Constant  OutDataTypeStr=single
  Divide : Product  Inputs=**
  Divide1 : Product  Inputs=**
  Divide2 : Product  Inputs=*/
  Memory : Memory  InitialCondition=1.75  InheritSampleTime=on
  Memory1 : Memory  InitialCondition=1.75  InheritSampleTime=on
  Saturation : Saturate  UpperLimit=10000  LowerLimit=1  OutDataTypeStr=single
      settings: AttributesFormatString="Min = %<LowerLimit>  Max = %<UpperLimit>"
  Switch : Switch  Criteria=u2 > Threshold
  Out : Outport
  wires:
  Add1/1 -> Switch/3
  Compare To Constant/1 -> Switch/2
  Abs/1 -> Compare To Constant/1
  Add3/1 -> Abs/1
  Memory1/1 -> Add3/2
  Constant1/1 -> Divide2/1
  Saturation/1 -> Divide2/2
  Memory/1 -> Divide1/2
  Divide2/1 -> Divide/2, Add2/1
  Switch/1 -> Out/1, Memory/1
  Divide1/1 -> Add1/2
  Add2/1 -> Divide1/1
  Constant/1 -> Add2/2
  Divide/1 -> Add1/1
  PtsNum/1 -> Saturation/1
  In/1 -> Divide/1, Add3/1, Switch/1, Memory1/1

== system MIL4L3_SW6_V1_20220211/CarMaker/VehicleControl/Function/LKA/LKAS1/LL/LL Inputs Mapping/bsLaneInfo/LanesReconstruct /RoadSide Offset/Road Width Calculation (RoadWCal)/Average Filter (AvrgFlt)1 ==
  In : Inport
  PtsNum : Inport  Port=2
  Add1 : Sum
  Add2 : Sum  Inputs=-+
  Constant : Constant  OutDataTypeStr=single
  Constant1 : Constant  OutDataTypeStr=single
  Divide : Product  Inputs=**
  Divide1 : Product  Inputs=**
  Divide2 : Product  Inputs=*/
  Memory : Memory  InitialCondition=3.2  InheritSampleTime=on
  Saturation : Saturate  UpperLimit=10000  LowerLimit=1  OutDataTypeStr=single
      settings: AttributesFormatString="Min = %<LowerLimit>  Max = %<UpperLimit>"
  Out : Outport
  wires:
  In/1 -> Divide/1
  PtsNum/1 -> Saturation/1
  Divide/1 -> Add1/1
  Constant/1 -> Add2/2
  Add2/1 -> Divide1/1
  Divide1/1 -> Add1/2
  Add1/1 -> Out/1, Memory/1
  Divide2/1 -> Add2/1, Divide/2
  Memory/1 -> Divide1/2
  Saturation/1 -> Divide2/2
  Constant1/1 -> Divide2/1

== system MIL4L3_SW6_V1_20220211/CarMaker/VehicleControl/Function/LKA/LKAS1/LL/LL Inputs Mapping/bsLaneInfo/LanesReconstruct /RoadSide Offset/Subsystem/Average Filter (AvrgFlt) ==
  In : Inport
  PtsNum : Inport  Port=2
  Abs : Abs
  Add1 : Sum  AccumDataTypeStr=single  OutDataTypeStr=single
  Add2 : Sum  Inputs=-+
  Add3 : Sum  Inputs=+-  AccumDataTypeStr=single  OutDataTypeStr=single
  Compare To Constant : simulink/Logic and Bit Operations/Compare To Constant  relop=>  const=0.5  OutDataTypeStr=boolean
  Constant : Constant  OutDataTypeStr=single
  Constant1 : Constant  OutDataTypeStr=single
  Divide : Product  Inputs=**
  Divide1 : Product  Inputs=**
  Divide2 : Product  Inputs=*/
  Memory : Memory  InitialCondition=-1.75  InheritSampleTime=on
  Memory1 : Memory  InitialCondition=-1.75  InheritSampleTime=on
  Saturation : Saturate  UpperLimit=10000  LowerLimit=1  OutDataTypeStr=single
      settings: AttributesFormatString="Min = %<LowerLimit>  Max = %<UpperLimit>"
  Switch : Switch  Criteria=u2 > Threshold
  Out : Outport
  wires:
  Add1/1 -> Switch/3
  Compare To Constant/1 -> Switch/2
  Abs/1 -> Compare To Constant/1
  Add3/1 -> Abs/1
  Memory1/1 -> Add3/2
  Constant1/1 -> Divide2/1
  Saturation/1 -> Divide2/2
  Memory/1 -> Divide1/2
  Divide2/1 -> Divide/2, Add2/1
  Switch/1 -> Out/1, Memory/1
  Divide1/1 -> Add1/2
  Add2/1 -> Divide1/1
  Constant/1 -> Add2/2
  Divide/1 -> Add1/1
  PtsNum/1 -> Saturation/1
  In/1 -> Divide/1, Add3/1, Switch/1, Memory1/1

== system MIL4L3_SW6_V1_20220211/CarMaker/VehicleControl/Function/LKA/LKAS1/LL/LLOn/LKA/LKA Motion Planning (LKAMP) /LKA Motion Planning Calculation (LKAMPCal)/Time Division (TDiv)/if action 1 ==
  In1 : Inport
  Action Port : ActionPort  InitializeStates=reset  ActionType=else
      settings: AttributesFormatString=states = %<InitializeStates>
  Out1 : Outport
      settings: AttributesFormatString=%<OutputWhenDisabled> = %<InitialOutput>
  wires:
  In1/1 -> Out1/1

== system MIL4L3_SW6_V1_20220211/CarMaker/VehicleControl/Function/LKA/LKAS1/LL/LLOn/LKA/LKA Motion Planning (LKAMP) /LKA Motion Planning Calculation (LKAMPCal)/Time Division (TDiv)/if action 2 ==
  Action Port : ActionPort  InitializeStates=reset  ActionType=then
      settings: AttributesFormatString=states = %<InitializeStates>
  Constant : Constant  Value=0  OutDataTypeStr=uint16
  Out1 : Outport
      settings: AttributesFormatString=%<OutputWhenDisabled> = %<InitialOutput>
  wires:
  Constant/1 -> Out1/1  "ModeFlg"

== system MIL4L3_SW6_V1_20220211/CarMaker/VehicleControl/Function/LKA/LKAS1/LL/LLOn/LKA/LKA Motion Planning (LKAMP) /LKA Motion Planning Calculation (LKAMPCal)/Time Division (TDiv)1/if action 3 ==
  In1 : Inport
  Action Port : ActionPort  InitializeStates=reset  ActionType=else
      settings: AttributesFormatString=states = %<InitializeStates>
  Out1 : Outport
      settings: AttributesFormatString=%<OutputWhenDisabled> = %<InitialOutput>
  wires:
  In1/1 -> Out1/1

== system MIL4L3_SW6_V1_20220211/CarMaker/VehicleControl/Function/LKA/LKAS1/LL/LLOn/LKA/LKA Motion Planning (LKAMP) /LKA Motion Planning Calculation (LKAMPCal)/Time Division (TDiv)1/if action 4 ==
  Action Port : ActionPort  InitializeStates=reset  ActionType=then
      settings: AttributesFormatString=states = %<InitializeStates>
  Constant : Constant  Value=0  OutDataTypeStr=single
  Out1 : Outport
      settings: AttributesFormatString=%<OutputWhenDisabled> = %<InitialOutput>
  wires:
  Constant/1 -> Out1/1  "ModeFlg"

== system MIL4L3_SW6_V1_20220211/CarMaker/VehicleControl/Function/LKA/LKAS1/LL/LLOn/LKA/LKA Motion Planning (LKAMP) /LKA Motion Planning Calculation (LKAMPCal)/Time Division (TDiv)2/if action 3 ==
  In1 : Inport
  Action Port : ActionPort  InitializeStates=reset  ActionType=else
      settings: AttributesFormatString=states = %<InitializeStates>
  Out1 : Outport
      settings: AttributesFormatString=%<OutputWhenDisabled> = %<InitialOutput>
  wires:
  In1/1 -> Out1/1

== system MIL4L3_SW6_V1_20220211/CarMaker/VehicleControl/Function/LKA/LKAS1/LL/LLOn/LKA/LKA Motion Planning (LKAMP) /LKA Motion Planning Calculation (LKAMPCal)/Time Division (TDiv)2/if action 4 ==
  Action Port : ActionPort  InitializeStates=reset  ActionType=then
      settings: AttributesFormatString=states = %<InitializeStates>
  Constant : Constant  Value=0  OutDataTypeStr=single
  Out1 : Outport
      settings: AttributesFormatString=%<OutputWhenDisabled> = %<InitialOutput>
  wires:
  Constant/1 -> Out1/1  "ModeFlg"

== system MIL4L3_SW6_V1_20220211/CarMaker/VehicleControl/Function/LKA/LKAS1/LL/LLOn/LKA/LKA Motion Planning (LKAMP) /LKA Motion Planning Calculation (LKAMPCal)/Time Division (TDiv)3/if action 3 ==
  In1 : Inport
  Action Port : ActionPort  InitializeStates=reset  ActionType=else
      settings: AttributesFormatString=states = %<InitializeStates>
  Out1 : Outport
      settings: AttributesFormatString=%<OutputWhenDisabled> = %<InitialOutput>
  wires:
  In1/1 -> Out1/1
